simulink model "Snap"  (R2024b)
settings: configuration reference "cigreConfig" (kept outside this file)
model workspace (MAT data in the model file):
  midSnapParamTop = Simulink.Parameter
  midSnapParamTop.Value = 3
  midSnapParamTop.Complexity = 'real'
  midSnapParamTop.Dimensions = [1 1]
  midSnapParamTop.DataType = 'int32'
  paramDouble = Simulink.Parameter
  paramDouble.Value = 6
  paramDouble.Complexity = 'real'
  paramDouble.Dimensions = [1 1]
  paramDouble.DataType = 'auto'
  paramInt = Simulink.Parameter
  paramInt.Value = 4
  paramInt.Complexity = 'real'
  paramInt.Dimensions = [1 1]
  paramInt.DataType = 'int32'
settings Model: DataDictionary=MySLDD.sldd  TunableVars=param  TunableVarsStorageClass=Auto  Creator=raarenst  LastModifiedBy=tomha
settings ConfigSetRef: SourceName=cigreConfig

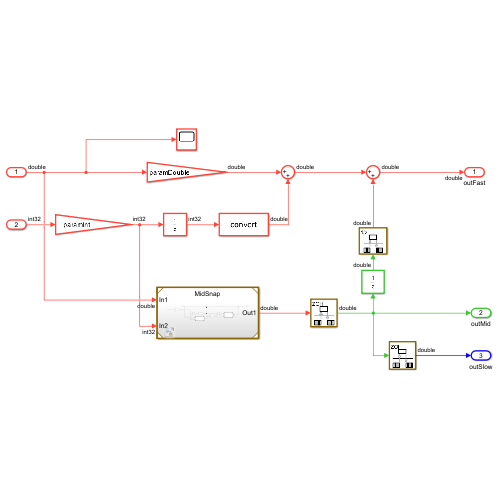
[thumbnail: Simulink's stored preview of the top-level diagram]
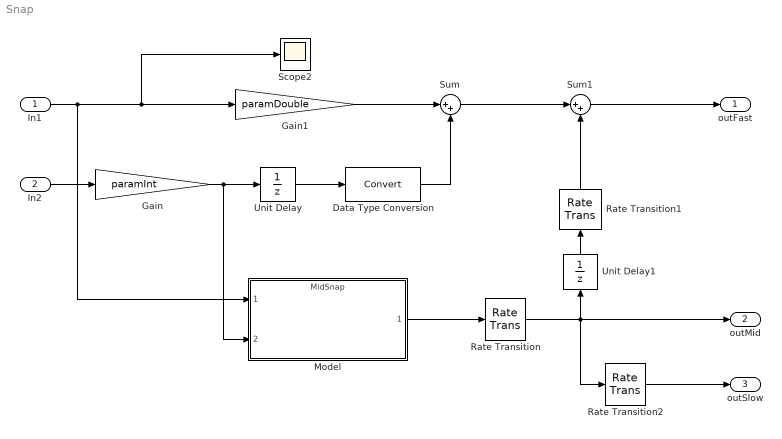
== system Snap ==
  In1 : Inport  OutDataTypeStr=double  SampleTime=0.1
  In2 : Inport  Port=2  OutDataTypeStr=int32  SampleTime=0.1
  Data Type Conversion : DataTypeConversion  SaturateOnIntegerOverflow=off  RndMeth=Floor
  Gain : Gain  Gain=paramInt  ParamDataTypeStr=int32  OutDataTypeStr=int32
  Gain1 : Gain  Gain=paramDouble  ParamDataTypeStr=double  OutDataTypeStr=Inherit: Same as input
  Model : ModelReference  ModelNameDialog=MidSnap  ParameterArgumentNames=midSnapParam  ParameterArgumentValues=midSnapParamTop  UsingDefaultArgumentValue=0  SimulationMode=Normal  ModelReferenceVersion=1.1
  Rate Transition : RateTransition  OutPortSampleTime=0.5
  Rate Transition1 : RateTransition  OutPortSampleTime=0.1
  Rate Transition2 : RateTransition  OutPortSampleTime=1
  Scope2 : Scope
  Sum : Sum  Inputs=|++
  Sum1 : Sum  Inputs=|++
  Unit Delay : UnitDelay  InitialCondition=3  SampleTime=-1  HasFrameUpgradeWarning=on
  Unit Delay1 : UnitDelay  InitialCondition=3  SampleTime=-1  HasFrameUpgradeWarning=on
  outFast : Outport  OutDataTypeStr=double
  outMid : Outport  Port=2
  outSlow : Outport  Port=3
  wires:
  In2/1 -> Gain/1
  Gain/1 -> Model/2, Unit Delay/1
  Unit Delay/1 -> Data Type Conversion/1
  In1/1 -> Model/1, Scope2/1, Gain1/1
  Data Type Conversion/1 -> Sum/2
  Model/1 -> Rate Transition/1
  Sum1/1 -> outFast/1
  Gain1/1 -> Sum/1
  Sum/1 -> Sum1/1
  Rate Transition/1 -> Rate Transition2/1, Unit Delay1/1, outMid/1
  Rate Transition1/1 -> Sum1/2
  Unit Delay1/1 -> Rate Transition1/1
  Rate Transition2/1 -> outSlow/1
